simulink model "task_A_All_mod"  (R2018a)
settings: Solver=ode45  StartTime=0.0  StopTime=10.0  RelTol=1e-3  EnableMultiTasking=on
values from neighbouring files (symbols this model uses):
  a0 = 8*lamda/(c*ro*(b-a)^2)    [task_A_scr.m]    (also in task_B_scr.m = 8*lamda/(3*c*ro*(b-a)^2); task_C_scr.m = 4*lamda*(2-A1-B1)/(c*ro*(b-a)^2))
  b0 = a0/2    [task_A_scr.m]    (also in task_B_scr.m)
  T_a = 350    [task_A_scr.m]    (also in task_C_scr.m = 600)
  T_b = 400    [task_A_scr.m]    (also in task_B_scr.m = 350; task_C_scr.m = 300)
undefined symbols (not defined in the file or in its folder): T_0
settings Model: Creator=Yurii  LastModifiedBy=Master
settings DataIOCC: LimitDataPoints=on  SaveFormat=Array
settings OptimizationCC: LifeSpan=inf
settings DebuggingCC: UnderspecifiedInitializationDetection=Classic  MergeDetectMultiDrivingBlocksExec=none  SolverPrmCheckMsg=warning  SFUnexpectedBacktrackingDiag=warning  SFNoUnconditionalDefaultTransitionDiag=warning  SFExecutionAtInitializationDiag=none
settings HardwareCC: ProdBitPerPointer=32  ProdBitPerSizeT=32  ProdBitPerPtrDiffT=32  ProdLargestAtomicFloat=None  ProdIntDivRoundTo=Undefined  ProdEndianess=Unspecified  ProdWordSize=32  ProdHWDeviceType=32-bit Generic
settings ModelReferenceCC: PropagateSignalLabelsOutOfModel=off
settings CodeAppCC: StateflowObjectComments=on
settings GRTTargetCC: TargetLangStandard=C89/C90 (ANSI)  GeneratePreprocessorConditionals=Disable all
settings ConfigComp: CovMetricSettings=dw  CovHtmlReporting=on  CovSaveCumulativeToWorkspaceVar=on  CovSaveSingleToWorkspaceVar=on  CovExternalEMLEnable=off

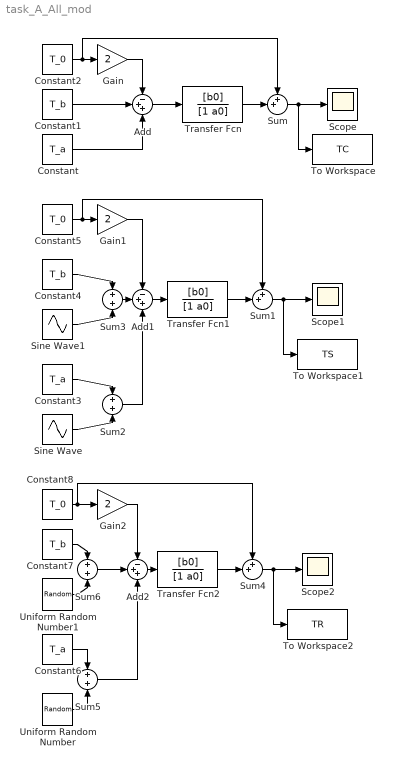
== system task_A_All_mod ==
  Add : Sum  Inputs=-++
  Add1 : Sum  Inputs=-++
  Add2 : Sum  Inputs=-++
  Constant : Constant  Value=T_a
  Constant1 : Constant  Value=T_b
  Constant2 : Constant  Value=T_0
  Constant3 : Constant  Value=T_a
  Constant4 : Constant  Value=T_b
  Constant5 : Constant  Value=T_0
  Constant6 : Constant  Value=T_a
  Constant7 : Constant  Value=T_b
  Constant8 : Constant  Value=T_0
  Gain : Gain  Gain=2
  Gain1 : Gain  Gain=2
  Gain2 : Gain  Gain=2
  Scope : Scope
  Scope1 : Scope
  Scope2 : Scope
  Sine Wave : Sin  Amplitude=0.05*T_a  SampleTime=0
  Sine Wave1 : Sin  Amplitude=0.05*T_b  SampleTime=0
  Sum : Sum  Inputs=++|
  Sum1 : Sum  Inputs=++|
  Sum{2..3,5..6} (4 alike) : Sum  Inputs=+|+
  Sum4 : Sum  Inputs=++|
  To Workspace : ToWorkspace  VariableName=TC  SaveFormat=Timeseries  SampleTime=-1
  To Workspace1 : ToWorkspace  VariableName=TS  SaveFormat=Timeseries  SampleTime=-1
  To Workspace2 : ToWorkspace  VariableName=TR  SaveFormat=Timeseries  SampleTime=-1
  Transfer Fcn : TransferFcn  Numerator=[b0]  Denominator=[1 a0]
  Transfer Fcn1 : TransferFcn  Numerator=[b0]  Denominator=[1 a0]
  Transfer Fcn2 : TransferFcn  Numerator=[b0]  Denominator=[1 a0]
  Uniform Random Number : UniformRandomNumber  Minimum=-0.05*T_a  Maximum=0.05*T_a  SampleTime=0.1
  Uniform Random Number1 : UniformRandomNumber  Minimum=-0.05*T_b  Maximum=0.05*T_b  SampleTime=0.1
  wires:
  Constant/1 -> Add/3
  Constant1/1 -> Add/2
  Constant2/1 -> Sum/1, Gain/1
  Gain/1 -> Add/1
  Add/1 -> Transfer Fcn/1
  Transfer Fcn/1 -> Sum/2
  Sum/1 -> To Workspace/1, Scope/1
  Sum3/1 -> Add1/2
  Constant5/1 -> Sum1/1, Gain1/1
  Sine Wave1/1 -> Sum3/2
  Constant3/1 -> Sum2/1
  Sine Wave/1 -> Sum2/2
  Sum1/1 -> To Workspace1/1, Scope1/1
  Transfer Fcn1/1 -> Sum1/2
  Sum2/1 -> Add1/3
  Add1/1 -> Transfer Fcn1/1
  Constant4/1 -> Sum3/1
  Gain1/1 -> Add1/1
  Sum6/1 -> Add2/2
  Sum4/1 -> To Workspace2/1, Scope2/1
  Uniform Random Number1/1 -> Sum6/2
  Sum5/1 -> Add2/3
  Uniform Random Number/1 -> Sum5/2
  Constant6/1 -> Sum5/1
  Transfer Fcn2/1 -> Sum4/2
  Gain2/1 -> Add2/1
  Constant7/1 -> Sum6/1
  Add2/1 -> Transfer Fcn2/1
  Constant8/1 -> Gain2/1, Sum4/1
